simulink model "model_sim"  (R2017b)
settings: Solver=FixedStepAuto  StartTime=0.0  StopTime=10  FixedStep=.001  RelTol=1e-3
settings Model: Creator=mariam  LastModifiedBy=mariam

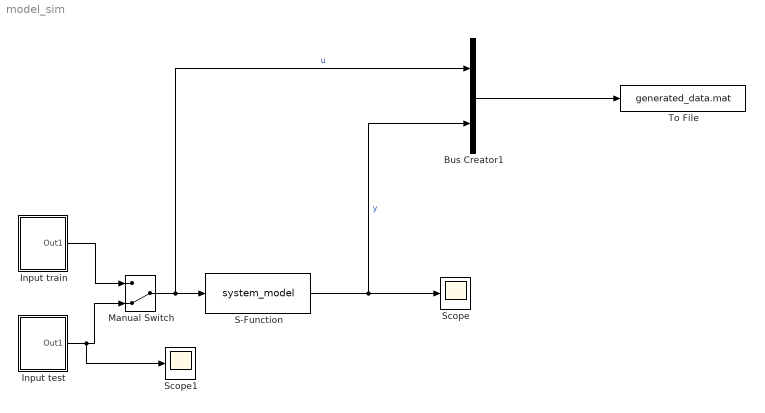
== system model_sim ==
  Bus Creator1 : BusCreator  Inputs=2
  Input test : Subsystem
  Input train : Subsystem
  Manual Switch : ManualSwitch  CurrentSetting=0
  S-Function : S-Function  FunctionName=system_model  SFunctionDeploymentMode=off  EnableBusSupport=off
  Scope : Scope
  Scope1 : Scope
  To File : ToFile  Filename=generated_data.mat  MatrixName=Inputs_Output
  wires:
  Manual Switch/1 -> Bus Creator1/1, S-Function/1  "u"
  S-Function/1 -> Bus Creator1/2, Scope/1  "y"
  Bus Creator1/1 -> To File/1
  Input train/1(Out1) -> Manual Switch/1
  Input test/1(Out1) -> Scope1/1, Manual Switch/2

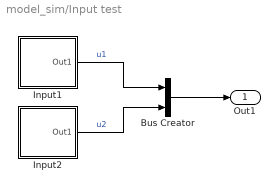
== system model_sim/Input test ==
  Bus Creator : BusCreator  Inputs=2
  Input1 : Subsystem
  Input2 : Subsystem
  Out1 : Outport
  wires:
  Input1/1(Out1) -> Bus Creator/1  "u1"
  Input2/1(Out1) -> Bus Creator/2  "u2"
  Bus Creator/1 -> Out1/1

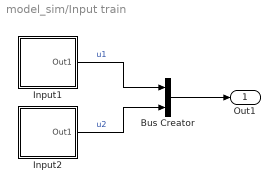
== system model_sim/Input train ==
  Bus Creator : BusCreator  Inputs=2
  Input1 : Subsystem
  Input2 : Subsystem
  Out1 : Outport
  wires:
  Bus Creator/1 -> Out1/1
  Input2/1(Out1) -> Bus Creator/2  "u2"
  Input1/1(Out1) -> Bus Creator/1  "u1"

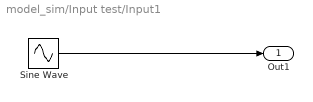
== system model_sim/Input test/Input1 ==
  Sine Wave : Sin  Amplitude=2  Frequency=12  SampleTime=0
  Out1 : Outport
  wires:
  Sine Wave/1 -> Out1/1

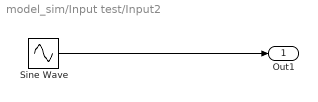
== system model_sim/Input test/Input2 ==
  Sine Wave : Sin  Amplitude=1.5  Frequency=20  SampleTime=0
  Out1 : Outport
  wires:
  Sine Wave/1 -> Out1/1

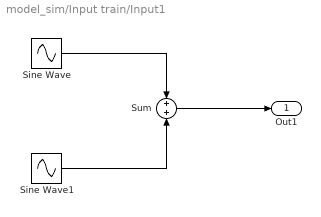
== system model_sim/Input train/Input1 ==
  Sine Wave : Sin  Frequency=2  SampleTime=0
  Sine Wave1 : Sin  Frequency=9  SampleTime=0
  Sum : Sum
  Out1 : Outport
  wires:
  Sine Wave1/1 -> Sum/2
  Sine Wave/1 -> Sum/1
  Sum/1 -> Out1/1

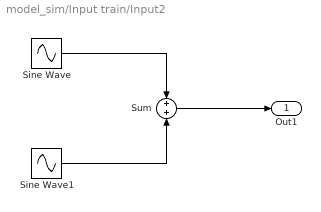
== system model_sim/Input train/Input2 ==
  Sine Wave : Sin  Frequency=6  SampleTime=0
  Sine Wave1 : Sin  Frequency=3  SampleTime=0
  Sum : Sum
  Out1 : Outport
  wires:
  Sum/1 -> Out1/1
  Sine Wave1/1 -> Sum/2
  Sine Wave/1 -> Sum/1
